simulink model "Program_Counter"  (R2024b)
settings: Solver=VariableStepAuto  StartTime=0.0  StopTime=10.0  RelTol=1e-3
settings Model: Creator=HP  LastModifiedBy=HP

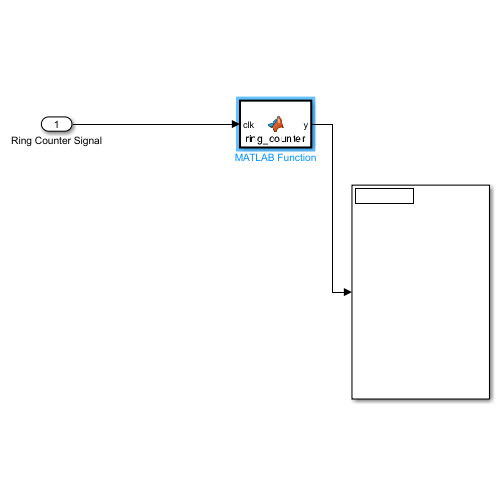
[thumbnail: Simulink's stored preview of the top-level diagram]
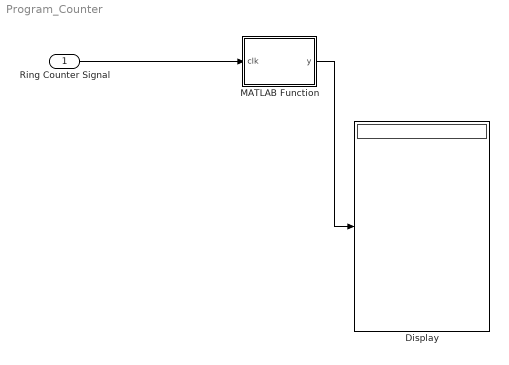
== system Program_Counter ==
  Ring Counter Signal : Inport
  Display : Display
  MATLAB Function : MATLAB Function  TreatAsAtomicUnit=on
  wires:
  MATLAB Function/1(y) -> Display/1
  Ring Counter Signal/1 -> MATLAB Function/1(clk)

== matlab function Program_Counter/MATLAB Function ==
  data: y output; clk input
function y = ring_counter(clk)
% 7-bit Ring Counter
persistent state
if isempty(state)
    state = [1 0 0 0 0 0 0]; % Initial state
end

if clk == 1
    state = circshift(state, [0 1]); % Shift right
end

y = state;
